simulink model "PlanarArmCLAug"  (R2025b)
settings: Solver=VariableStepAuto  StartTime=0.0  StopTime=10.0  RelTol=1e-3
undefined symbols (not defined in the file): JacobuInv, Kp, Kv, uss
libraries: RCTblocks x2, cstblocks x1
settings Model: Creator=d.alazard  LastModifiedBy=andre
settings SolverCC: AlgebraicLoopSolver=TrustRegion
settings DebuggingCC: AlgebraicLoopMsg=none  UnconnectedInputMsg=warning  UnconnectedOutputMsg=warning  UnconnectedLineMsg=warning
settings ModelReferenceCC: EnableRefExpFcnMdlSchedulingChecks=on
settings RTWCC: GPUComputeCapability=3.5  DLArmComputeVersion=19.05

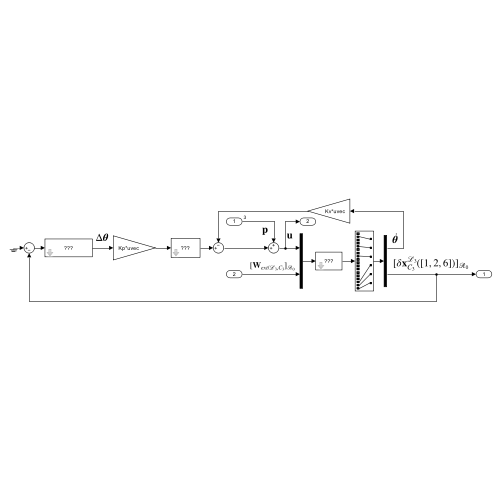
[thumbnail: Simulink's stored preview of the top-level diagram]
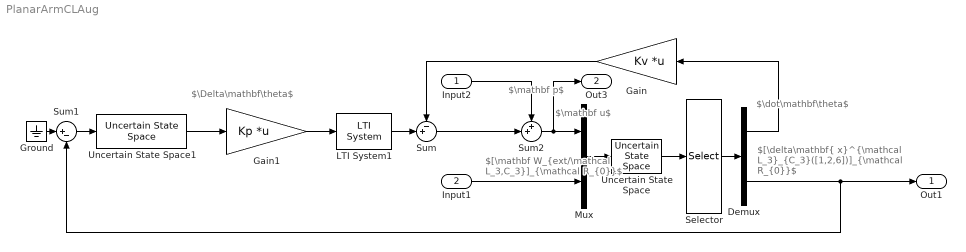
== system PlanarArmCLAug ==
  note: $[\delta\mathbf{ x}^{\mathcal L_3}_{C_3}([1,2,6])]_{\mathcal R_{0}}$
  note: $\dot\mathbf\theta$
  note: $\mathbf u$
  note: $\Delta\mathbf\theta$
  note: $[\mathbf W_{ext/\mathcal L_3,C_3}]_{\mathcal R_{0}}$
  note: $\mathbf p$
  Input2 : Inport  OutDataTypeStr=uint64  PortDimensions=3
  Input1 : Inport  Port=2
  Demux : Demux  Outputs=[3 3]
  Gain : Gain  Gain=Kv  Multiplication=Matrix(K*u) (u vector)
  Gain1 : Gain  Gain=Kp  Multiplication=Matrix(K*u) (u vector)
  Ground : Ground
  LTI System1 : cstblocks/LTI System  sys=F  IC=[]  PadeOrder=0
  Mux : Mux  Inputs=[3 3]
  Selector : Selector  InputPortWidth=18  IndexOptions=Index vector (dialog)  Indices=[2 5 8 16 17 18]  OutputSizes=1
  Sum : Sum  Inputs=-+|
  Sum1 : Sum  Inputs=|+-
  Sum2 : Sum  Inputs=++|
  Uncertain State Space : RCTblocks/Uncertain State Space  Tag=USS  USystem=Gfu  UValue=[]  X0=[]  uX0=[]
  Uncertain State Space1 : RCTblocks/Uncertain State Space  Tag=USS  USystem=uss(JacobuInv)  UValue=[]  X0=[]  uX0=[]
  Out1 : Outport
  Out3 : Outport  Port=2
  wires:
  Demux/1 -> Gain/1
  Gain/1 -> Sum/1
  Ground/1 -> Sum1/1
  Demux/2 -> Out1/1, Sum1/2
  Uncertain State Space1/1 -> Gain1/1
  Sum1/1 -> Uncertain State Space1/1
  Mux/1 -> Uncertain State Space/1
  Input1/1 -> Mux/2
  Sum/1 -> Sum2/2
  Sum2/1 -> Out3/1, Mux/1
  Input2/1 -> Sum2/1
  Gain1/1 -> LTI System1/1
  LTI System1/1 -> Sum/2
  Uncertain State Space/1 -> Selector/1
  Selector/1 -> Demux/1
